simulink model "FWBridgeRectifier"  (R2018b)
settings: Solver=ode45  StartTime=0.0  StopTime=0.05  RelTol=1e-3  EnableMultiTasking=on
libraries: fl_lib x7, elec_lib x4, rftxlines1 x2, rfseriesshuntrlcs1 x1
settings Model: Creator=MuhammadHarris  LastModifiedBy=rishhanth
settings DataIOCC: LimitDataPoints=on  SaveFormat=Array
settings OptimizationCC: LifeSpan=inf
settings DebuggingCC: SolverPrmCheckMsg=warning  SFUnexpectedBacktrackingDiag=warning  SFNoUnconditionalDefaultTransitionDiag=warning  SFExecutionAtInitializationDiag=none
settings HardwareCC: ProdBitPerPointer=32  ProdBitPerSizeT=32  ProdBitPerPtrDiffT=32  ProdLargestAtomicFloat=None  ProdIntDivRoundTo=Undefined  ProdEndianess=Unspecified  ProdWordSize=32  ProdHWDeviceType=32-bit Generic
settings ModelReferenceCC: PropagateSignalLabelsOutOfModel=off
settings SFSimCC: SimUseLocalCustomCode=off
settings RTWCC: RTWUseLocalCustomCode=off
settings CodeAppCC: StateflowObjectComments=on
settings GRTTargetCC: TargetLangStandard=C89/C90 (ANSI)  GeneratePreprocessorConditionals=Disable all
settings ConfigComp: CovMetricSettings=dw  CovHtmlReporting=on  CovSaveCumulativeToWorkspaceVar=on  CovSaveSingleToWorkspaceVar=on  CovExternalEMLEnable=off  CovSFcnEnable=off
settings SimscapeCC: SimscapeNormalizeSystem=off

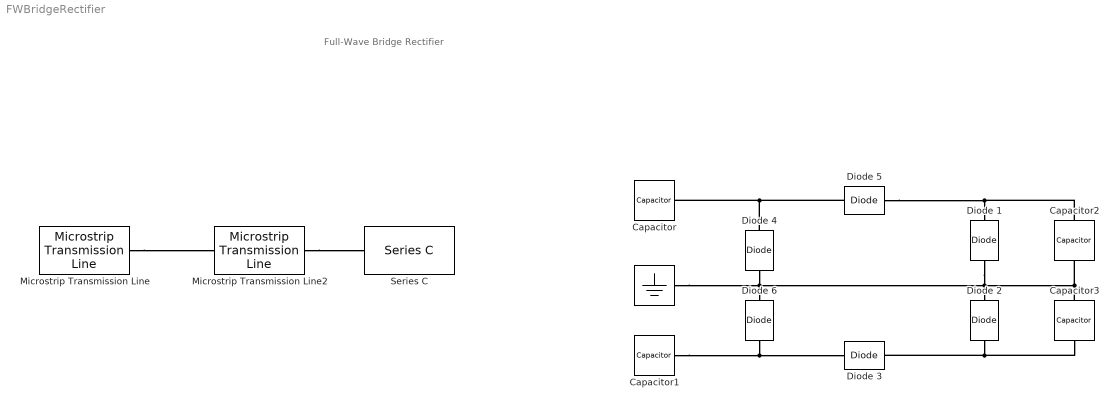
== system FWBridgeRectifier ==
  note: Full-Wave Bridge Rectifier
  " " : fl_lib/Electrical/Electrical Elements/Electrical Reference
  Capacitor{,1..3} (4 alike) : elec_lib/Passive Devices/Capacitor  enable_table=0  c=1e-6 F  Cvec=[1e-05, 1e-06] F  Vvec=[0, 10] V  CV_table_symmetry=1  C_tol=5  enable_C_tol=0  tol_distribution=1  nSigma=4  r=1e-6 Ohm  g=0 1/Ohm  enable_operating_limits=0  operating_limit_action=2  max_working_voltage_range=[-25, 25] V  power_rating=1 W  enable_faults=0  fault_action=1  Cscale_faulted=100  R_faulted=1e-3 Ohm  G_faulted=0 1/Ohm  tau_fault=1e-3 s  enable_temporal_fault=0  t_fault=1 s  enable_behavioral_fault=0  max_permissible_voltage_range=[-100, 100] V  t_fail_on_voltage=1 s  i_specify=off  i_priority=None  i=0 A  i_nominal_specify=off  i_nominal_unit=A  i_nominal_value=1  v_specify=off  v_priority=None  v=0 V  v_nominal_specify=off  v_nominal_unit=V  v_nominal_value=1  vc_specify=off  vc_priority=High  vc=0 V  vc_nominal_specify=off  vc_nominal_unit=V  vc_nominal_value=1
  Diode {1..6} (6 alike) : fl_lib/Electrical/Electrical Elements/Diode  Vf=0.7 V  Ron=0.3 Ohm  Goff=1e-8 1/Ohm  i_specify=off  i_priority=High  i=0 A  i_nominal_specify=off  i_nominal_unit=A  i_nominal_value=1  v_specify=off  v_priority=High  v=0 V  v_nominal_specify=off  v_nominal_unit=V  v_nominal_value=1
  Microstrip Transmission Line : rftxlines1/Microstrip Transmission Line  LConnTagsString=__newl0  RConnTagsString=__newr0  Width=2e-3  Height=0.635e-3  Thickness=0.005e-3  EpsilonR=9.8  LossTangent=0  SigmaCond=inf  LineLength=10e-3  StubMode=Series  Termination=Short  PlotFreq=User-specified  SourceFreq=User-specified  Freq=[1e9:1.0e6:3e9]  AllPlotType=X-Y plane  AppliedNetworkData=S21  AppliedComplexFormat=Angle (degrees)  AppliedNetworkData2=S11  AppliedComplexFormat2=Magnitude (decibels)  AppliedXParameter=Freq  AppliedXFormat=Auto  YOption=Linear  XOption=Linear  PlotZ0=50  DisplayData=off  PlotFreqNoSim=User-specified  NetworkData=S21  SmithData=S11  PolarData=S11  ComplexFormat=Angle  DBFormat=Magnitude (decibels)  NoneFormat=None
      settings: SourceProductName=RF Blockset  SourceProductBaseCode=RB
  Microstrip Transmission Line2 : rftxlines1/Microstrip Transmission Line  LConnTagsString=__newl0  RConnTagsString=__newr0  Width=2e-3  Height=0.635e-3  Thickness=0.005e-3  EpsilonR=9.8  LossTangent=0  SigmaCond=inf  LineLength=26.3e-3  StubMode=Series  Termination=Short  PlotFreq=User-specified  SourceFreq=User-specified  Freq=[1e9:1.0e6:3e9]  AllPlotType=X-Y plane  AppliedNetworkData=S21  AppliedComplexFormat=Angle (degrees)  AppliedNetworkData2=S11  AppliedComplexFormat2=Magnitude (decibels)  AppliedXParameter=Freq  AppliedXFormat=Auto  YOption=Linear  XOption=Linear  PlotZ0=50  DisplayData=off  PlotFreqNoSim=User-specified  NetworkData=S21  SmithData=S11  PolarData=S11  ComplexFormat=Angle  DBFormat=Magnitude (decibels)  NoneFormat=None
      settings: SourceProductName=RF Blockset  SourceProductBaseCode=RB
  Series C : rfseriesshuntrlcs1/Series C  LConnTagsString=__newl0  RConnTagsString=__newr0  R=0  L=0  C=1e-12  PlotFreq=User-specified  SourceFreq=User-specified  Freq=[1:1.0e5:4e6]  AllPlotType=X-Y plane  AppliedNetworkData=S21  AppliedComplexFormat=Magnitude (decibels)  AppliedNetworkData2=""  AppliedXParameter=Freq  AppliedXFormat=Hz  YOption=Linear  XOption=Linear  PlotZ0=50  DisplayData=off  PlotFreqNoSim=User-specified  NetworkData=S21  SmithData=S11  PolarData=S11  ComplexFormat=Magnitude (decibels)  DBFormat=Magnitude (decibels)  NoneFormat=None
      settings: SourceProductName=RF Blockset  SourceProductBaseCode=RB
  connections:
  Diode 5/LConn1 -- Diode 4/RConn1 -- Capacitor/RConn1
  Diode 5/RConn1 -- Capacitor2/LConn1 -- Diode 1/RConn1
  Diode 2/LConn1 -- Capacitor3/RConn1 -- Diode 3/LConn1
  Diode 6/LConn1 -- Capacitor1/RConn1 -- Diode 3/RConn1
  Diode 4/LConn1 -- " "/LConn1 -- Diode 1/LConn1 -- Capacitor3/LConn1 -- Capacitor2/RConn1 -- Diode 2/RConn1 -- Diode 6/RConn1
  Microstrip Transmission Line/RConn1 -- Microstrip Transmission Line2/LConn1
  Microstrip Transmission Line2/RConn1 -- Series C/LConn1
